simulink model "projekt"  (R2021b)
settings: Solver=FixedStepAuto  StartTime=0.0  StopTime=Inf  RelTol=1e-3  EnableMultiTasking=on
libraries: c2837xDlib x30
settings Model: ExtModeTrigDuration=8  Creator=gabrys  LastModifiedBy=gabrys
settings SolverCC: AutoInsertRateTranBlk=on
settings OptimizationCC: DefaultUnderspecifiedDataType=single  EnhancedBackFolding=on  PassReuseOutputArgsAs=Individual arguments  MaxStackSize=1024  OptimizeBlockOrder=speed  DifferentSizesBufferReuse=on  OptimizationCustomize=off  DenormalBehavior=FlushToZero  EfficientTunableParamExpr=on
settings DebuggingCC: ParameterTunabilityLossMsg=error
settings HardwareCC: ProdBitPerChar=16  ProdBitPerInt=16  ProdBitPerPointer=32  ProdBitPerSizeT=32  ProdBitPerPtrDiffT=32  ProdLargestAtomicInteger=Integer  ProdLargestAtomicFloat=None  ProdWordSize=16  ProdLongLongMode=on  ProdHWDeviceType=Texas Instruments->C2000
settings ModelReferenceCC: ModelReferenceNumInstancesAllowed=Single
settings SFSimCC: MATLABDynamicMemAlloc=off
settings RTWCC: Description=Embedded Coder  SystemTargetFile=ert.tlc  HardwareBoard=TI Delfino F28379D LaunchPad  TemplateMakefile=ert_default_tmf  Toolchain=Texas Instruments Code Composer Studio (C2000)
settings CodeAppCC: ForceParamTrailComments=on  IgnoreCustomStorageClasses=off  OperatorAnnotations=on  SimulinkDataObjDesc=on  SFDataObjDesc=on  InsertBlockDesc=on
settings ERTTargetCC: CodeReplacementLibrary=TI C28x  ExtModeTransport=4  ExtModeStaticAlloc=on  ExtModeMexFile=ext_xcp  ExtModeIntrfLevel=Level2 - Open

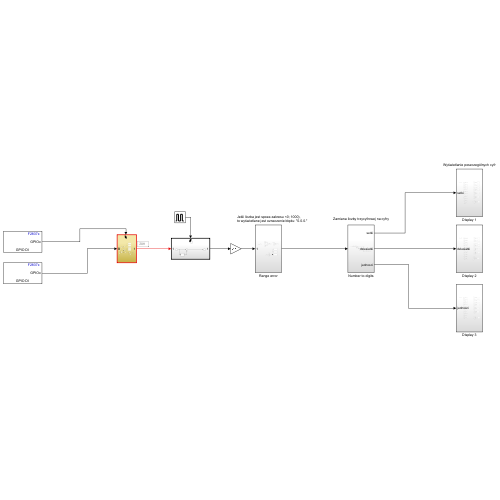
[thumbnail: Simulink's stored preview of the top-level diagram]
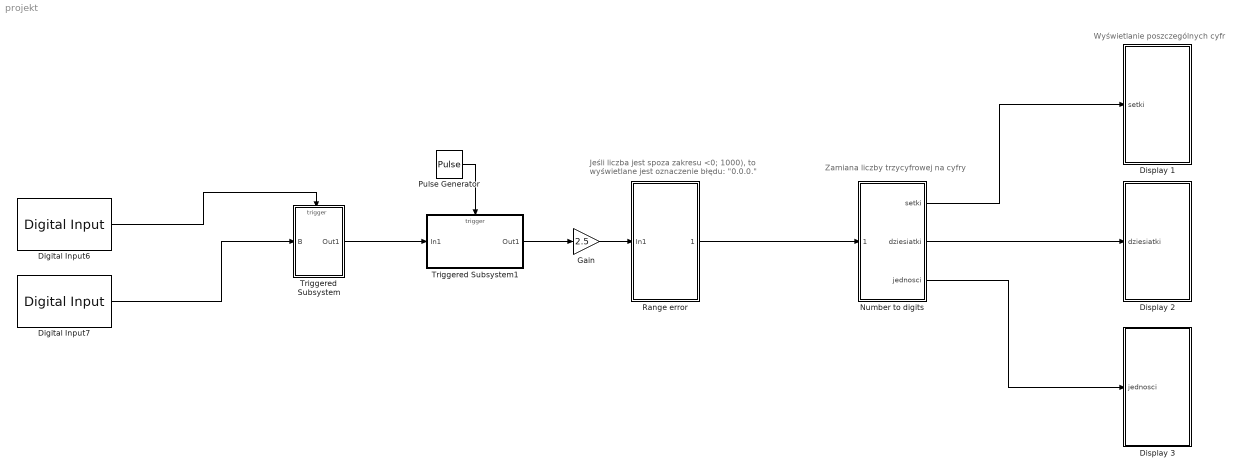
== system projekt ==
  note: Jeśli liczba jest spoza zakresu <0; 1000),
      | to wyświetlane jest oznaczenie błędu: "0.0.0."
  note: Wyświetlanie poszczególnych cyfr
  note: Zamiana liczby trzycyfrowej na cyfry
  Digital Input6 : c2837xDlib/Digital Input  GPIO_Number=GPIO128~GPIO135  GPIO_Bit0=off  GPIO_Bit1=off  GPIO_Bit2=on  GPIO_Bit3=off  GPIO_Bit4=off  GPIO_Bit5=off  GPIO_Bit6=off  GPIO_Bit7=off  sampleTime=0.01  dataType=auto  GPIO_Bit0_Qualification=Sync to SYSCLKOUT  GPIO_Bit1_Qualification=Sync to SYSCLKOUT  GPIO_Bit2_Qualification=Sync to SYSCLKOUT  GPIO_Bit3_Qualification=Sync to SYSCLKOUT  GPIO_Bit4_Qualification=Sync to SYSCLKOUT  GPIO_Bit5_Qualification=Sync to SYSCLKOUT  GPIO_Bit6_Qualification=Sync to SYSCLKOUT  GPIO_Bit7_Qualification=Sync to SYSCLKOUT  Qualification_Period=-1
      settings: SourceProductBaseCode=TIC2000
  Digital Input7 : c2837xDlib/Digital Input  GPIO_Number=GPIO128~GPIO135  GPIO_Bit0=off  GPIO_Bit1=off  GPIO_Bit2=off  GPIO_Bit3=on  GPIO_Bit4=off  GPIO_Bit5=off  GPIO_Bit6=off  GPIO_Bit7=off  sampleTime=0.01  dataType=auto  GPIO_Bit0_Qualification=Sync to SYSCLKOUT  GPIO_Bit1_Qualification=Sync to SYSCLKOUT  GPIO_Bit2_Qualification=Sync to SYSCLKOUT  GPIO_Bit3_Qualification=Sync to SYSCLKOUT  GPIO_Bit4_Qualification=Sync to SYSCLKOUT  GPIO_Bit5_Qualification=Sync to SYSCLKOUT  GPIO_Bit6_Qualification=Sync to SYSCLKOUT  GPIO_Bit7_Qualification=Sync to SYSCLKOUT  Qualification_Period=-1
      settings: SourceProductBaseCode=TIC2000
  Display 1 : Subsystem
  Display 2 : Subsystem
  Display 3 : Subsystem
  Gain : Gain  Gain=2.5
  Number to digits : Subsystem
  Pulse Generator : DiscretePulseGenerator  PulseType=Time based  Period=1  PulseWidth=50
  Range error : Subsystem
  Triggered Subsystem : Subsystem  TreatAsAtomicUnit=on
  Triggered Subsystem1 : Subsystem  TreatAsAtomicUnit=on
  wires:
  Number to digits/3(jednosci) -> Display 3/1(jednosci)
  Range error/1(" ") -> Number to digits/1(" ")
  Number to digits/2(dziesiatki) -> Display 2/1(dziesiatki)
  Number to digits/1(setki) -> Display 1/1(setki)
  Digital Input7/1 -> Triggered Subsystem/1(B)
  Digital Input6/1 -> Triggered Subsystem/Trigger
  Pulse Generator/1 -> Triggered Subsystem1/Trigger
  Triggered Subsystem1/1(Out1) -> Gain/1
  Gain/1 -> Range error/1(In1)
  Triggered Subsystem/1(Out1) -> Triggered Subsystem1/1(In1)

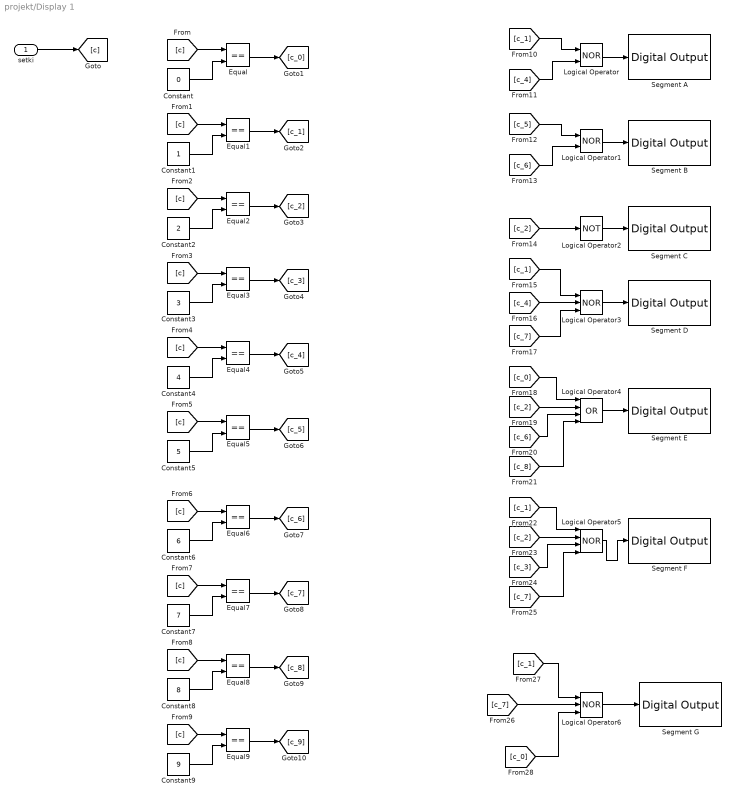
== system projekt/Display 1 ==
  setki : Inport
  Constant : Constant  Value=0
  Constant1 : Constant
  Constant2 : Constant  Value=2
  Constant3 : Constant  Value=3
  Constant4 : Constant  Value=4
  Constant5 : Constant  Value=5
  Constant6 : Constant  Value=6
  Constant7 : Constant  Value=7
  Constant8 : Constant  Value=8
  Constant9 : Constant  Value=9
  Equal{,1..9} (10 alike) : RelationalOperator  Operator===  OutDataTypeStr=boolean  RndMeth=Simplest
  Logical Operator : Logic  Operator=NOR  AllPortsSameDT=off  OutDataTypeStr=boolean
  Logical Operator1 : Logic  Operator=NOR  AllPortsSameDT=off  OutDataTypeStr=boolean
  Logical Operator2 : Logic  Operator=NOT  AllPortsSameDT=off  OutDataTypeStr=boolean
  Logical Operator3 : Logic  Operator=NOR  Inputs=3  AllPortsSameDT=off  OutDataTypeStr=boolean
  Logical Operator4 : Logic  Operator=OR  Inputs=4  AllPortsSameDT=off  OutDataTypeStr=boolean
  Logical Operator5 : Logic  Operator=NOR  Inputs=4  AllPortsSameDT=off  OutDataTypeStr=boolean
  Logical Operator6 : Logic  Operator=NOR  Inputs=3  AllPortsSameDT=off  OutDataTypeStr=boolean
  Segment A : c2837xDlib/Digital Output  GPIO_Number=GPIO0~GPIO7  GPIO_Bit0=off  GPIO_BIT0_Toggle=off  GPIO_Bit1=on  GPIO_BIT1_Toggle=off  GPIO_Bit2=off  GPIO_BIT2_Toggle=off  GPIO_Bit3=off  GPIO_BIT3_Toggle=off  GPIO_Bit4=off  GPIO_BIT4_Toggle=off  GPIO_Bit5=off  GPIO_BIT5_Toggle=off  GPIO_Bit6=off  GPIO_BIT6_Toggle=off  GPIO_Bit7=off  GPIO_BIT7_Toggle=off
      settings: SourceProductBaseCode=TIC2000
  Segment B : c2837xDlib/Digital Output  GPIO_Number=GPIO120~GPIO127  GPIO_Bit0=off  GPIO_BIT0_Toggle=off  GPIO_Bit1=off  GPIO_BIT1_Toggle=off  GPIO_Bit2=off  GPIO_BIT2_Toggle=off  GPIO_Bit3=on  GPIO_BIT3_Toggle=off  GPIO_Bit4=off  GPIO_BIT4_Toggle=off  GPIO_Bit5=off  GPIO_BIT5_Toggle=off  GPIO_Bit6=off  GPIO_BIT6_Toggle=off  GPIO_Bit7=off  GPIO_BIT7_Toggle=off
      settings: SourceProductBaseCode=TIC2000
  Segment C : c2837xDlib/Digital Output  GPIO_Number=GPIO16~GPIO23  GPIO_Bit0=off  GPIO_BIT0_Toggle=off  GPIO_Bit1=off  GPIO_BIT1_Toggle=off  GPIO_Bit2=on  GPIO_BIT2_Toggle=off  GPIO_Bit3=off  GPIO_BIT3_Toggle=off  GPIO_Bit4=off  GPIO_BIT4_Toggle=off  GPIO_Bit5=off  GPIO_BIT5_Toggle=off  GPIO_Bit6=off  GPIO_BIT6_Toggle=off  GPIO_Bit7=off  GPIO_BIT7_Toggle=off
      settings: SourceProductBaseCode=TIC2000
  Segment D : c2837xDlib/Digital Output  GPIO_Number=GPIO16~GPIO23  GPIO_Bit0=off  GPIO_BIT0_Toggle=off  GPIO_Bit1=off  GPIO_BIT1_Toggle=off  GPIO_Bit2=off  GPIO_BIT2_Toggle=off  GPIO_Bit3=on  GPIO_BIT3_Toggle=off  GPIO_Bit4=off  GPIO_BIT4_Toggle=off  GPIO_Bit5=off  GPIO_BIT5_Toggle=off  GPIO_Bit6=off  GPIO_BIT6_Toggle=off  GPIO_Bit7=off  GPIO_BIT7_Toggle=off
      settings: SourceProductBaseCode=TIC2000
  Segment E : c2837xDlib/Digital Output  GPIO_Number=GPIO32~GPIO39  GPIO_Bit0=on  GPIO_BIT0_Toggle=off  GPIO_Bit1=off  GPIO_BIT1_Toggle=off  GPIO_Bit2=off  GPIO_BIT2_Toggle=off  GPIO_Bit3=off  GPIO_BIT3_Toggle=off  GPIO_Bit4=off  GPIO_BIT4_Toggle=off  GPIO_Bit5=off  GPIO_BIT5_Toggle=off  GPIO_Bit6=off  GPIO_BIT6_Toggle=off  GPIO_Bit7=off  GPIO_BIT7_Toggle=off
      settings: SourceProductBaseCode=TIC2000
  Segment F : c2837xDlib/Digital Output  GPIO_Number=GPIO56~GPIO63  GPIO_Bit0=off  GPIO_BIT0_Toggle=off  GPIO_Bit1=off  GPIO_BIT1_Toggle=off  GPIO_Bit2=off  GPIO_BIT2_Toggle=off  GPIO_Bit3=off  GPIO_BIT3_Toggle=off  GPIO_Bit4=off  GPIO_BIT4_Toggle=off  GPIO_Bit5=on  GPIO_BIT5_Toggle=off  GPIO_Bit6=off  GPIO_BIT6_Toggle=off  GPIO_Bit7=off  GPIO_BIT7_Toggle=off
      settings: SourceProductBaseCode=TIC2000
  Segment G : c2837xDlib/Digital Output  GPIO_Number=GPIO0~GPIO7  GPIO_Bit0=on  GPIO_BIT0_Toggle=off  GPIO_Bit1=off  GPIO_BIT1_Toggle=off  GPIO_Bit2=off  GPIO_BIT2_Toggle=off  GPIO_Bit3=off  GPIO_BIT3_Toggle=off  GPIO_Bit4=off  GPIO_BIT4_Toggle=off  GPIO_Bit5=off  GPIO_BIT5_Toggle=off  GPIO_Bit6=off  GPIO_BIT6_Toggle=off  GPIO_Bit7=off  GPIO_BIT7_Toggle=off
      settings: SourceProductBaseCode=TIC2000
  wires:
  setki/1 -> [c]
  [c] -> Equal/1
  Constant/1 -> Equal/2
  Equal/1 -> [c_0]
  Constant1/1 -> Equal1/2
  [c] -> Equal1/1
  Equal1/1 -> [c_1]
  Constant2/1 -> Equal2/2
  [c] -> Equal2/1
  Equal2/1 -> [c_2]
  Equal4/1 -> [c_4]
  Constant4/1 -> Equal4/2
  [c] -> Equal4/1
  [c] -> Equal5/1
  Constant5/1 -> Equal5/2
  Constant3/1 -> Equal3/2
  [c] -> Equal3/1
  Equal3/1 -> [c_3]
  Equal5/1 -> [c_5]
  Equal6/1 -> [c_6]
  Constant6/1 -> Equal6/2
  Equal7/1 -> [c_7]
  [c] -> Equal7/1
  [c] -> Equal6/1
  Constant7/1 -> Equal7/2
  [c] -> Equal8/1
  Constant8/1 -> Equal8/2
  [c] -> Equal9/1
  Constant9/1 -> Equal9/2
  Equal8/1 -> [c_8]
  Equal9/1 -> [c_9]
  Logical Operator/1 -> Segment A/1
  [c_1] -> Logical Operator/1
  [c_4] -> Logical Operator/2
  [c_6] -> Logical Operator1/2
  Logical Operator1/1 -> Segment B/1
  [c_5] -> Logical Operator1/1
  [c_2] -> Logical Operator2/1
  Logical Operator2/1 -> Segment C/1
  [c_1] -> Logical Operator3/1
  Logical Operator3/1 -> Segment D/1
  [c_4] -> Logical Operator3/2
  [c_7] -> Logical Operator3/3
  [c_6] -> Logical Operator4/3
  [c_2] -> Logical Operator4/2
  Logical Operator4/1 -> Segment E/1
  [c_0] -> Logical Operator4/1
  [c_8] -> Logical Operator4/4
  [c_2] -> Logical Operator5/2
  [c_1] -> Logical Operator5/1
  Logical Operator5/1 -> Segment F/1
  [c_3] -> Logical Operator5/3
  [c_7] -> Logical Operator5/4
  [c_7] -> Logical Operator6/2
  Logical Operator6/1 -> Segment G/1
  [c_1] -> Logical Operator6/1
  [c_0] -> Logical Operator6/3

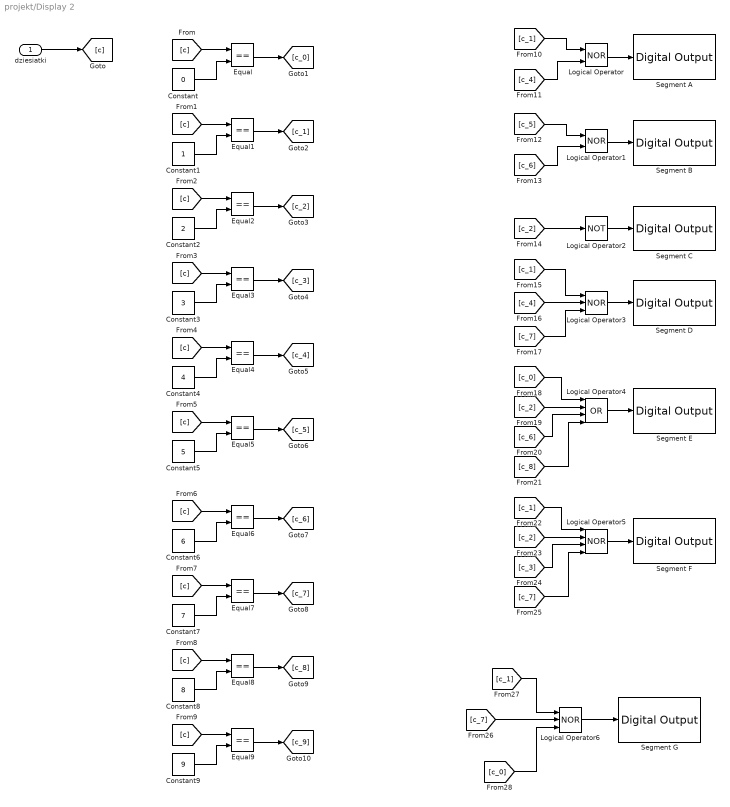
== system projekt/Display 2 ==
  dziesiatki : Inport
  Constant : Constant  Value=0
  Constant1 : Constant
  Constant2 : Constant  Value=2
  Constant3 : Constant  Value=3
  Constant4 : Constant  Value=4
  Constant5 : Constant  Value=5
  Constant6 : Constant  Value=6
  Constant7 : Constant  Value=7
  Constant8 : Constant  Value=8
  Constant9 : Constant  Value=9
  Equal{,1..9} (10 alike) : RelationalOperator  Operator===  OutDataTypeStr=boolean  RndMeth=Simplest
  Logical Operator : Logic  Operator=NOR  AllPortsSameDT=off  OutDataTypeStr=boolean
  Logical Operator1 : Logic  Operator=NOR  AllPortsSameDT=off  OutDataTypeStr=boolean
  Logical Operator2 : Logic  Operator=NOT  AllPortsSameDT=off  OutDataTypeStr=boolean
  Logical Operator3 : Logic  Operator=NOR  Inputs=3  AllPortsSameDT=off  OutDataTypeStr=boolean
  Logical Operator4 : Logic  Operator=OR  Inputs=4  AllPortsSameDT=off  OutDataTypeStr=boolean
  Logical Operator5 : Logic  Operator=NOR  Inputs=4  AllPortsSameDT=off  OutDataTypeStr=boolean
  Logical Operator6 : Logic  Operator=NOR  Inputs=3  AllPortsSameDT=off  OutDataTypeStr=boolean
  Segment A : c2837xDlib/Digital Output  GPIO_Number=GPIO120~GPIO127  GPIO_Bit0=off  GPIO_BIT0_Toggle=off  GPIO_Bit1=off  GPIO_BIT1_Toggle=off  GPIO_Bit2=on  GPIO_BIT2_Toggle=off  GPIO_Bit3=off  GPIO_BIT3_Toggle=off  GPIO_Bit4=off  GPIO_BIT4_Toggle=off  GPIO_Bit5=off  GPIO_BIT5_Toggle=off  GPIO_Bit6=off  GPIO_BIT6_Toggle=off  GPIO_Bit7=off  GPIO_BIT7_Toggle=off
      settings: SourceProductBaseCode=TIC2000
  Segment B : c2837xDlib/Digital Output  GPIO_Number=GPIO0~GPIO7  GPIO_Bit0=off  GPIO_BIT0_Toggle=off  GPIO_Bit1=off  GPIO_BIT1_Toggle=off  GPIO_Bit2=off  GPIO_BIT2_Toggle=off  GPIO_Bit3=off  GPIO_BIT3_Toggle=off  GPIO_Bit4=on  GPIO_BIT4_Toggle=off  GPIO_Bit5=off  GPIO_BIT5_Toggle=off  GPIO_Bit6=off  GPIO_BIT6_Toggle=off  GPIO_Bit7=off  GPIO_BIT7_Toggle=off
      settings: SourceProductBaseCode=TIC2000
  Segment C : c2837xDlib/Digital Output  GPIO_Number=GPIO16~GPIO23  GPIO_Bit0=off  GPIO_BIT0_Toggle=off  GPIO_Bit1=off  GPIO_BIT1_Toggle=off  GPIO_Bit2=off  GPIO_BIT2_Toggle=off  GPIO_Bit3=off  GPIO_BIT3_Toggle=off  GPIO_Bit4=off  GPIO_BIT4_Toggle=off  GPIO_Bit5=off  GPIO_BIT5_Toggle=off  GPIO_Bit6=on  GPIO_BIT6_Toggle=off  GPIO_Bit7=off  GPIO_BIT7_Toggle=off
      settings: SourceProductBaseCode=TIC2000
  Segment D : c2837xDlib/Digital Output  GPIO_Number=GPIO56~GPIO63  GPIO_Bit0=off  GPIO_BIT0_Toggle=off  GPIO_Bit1=off  GPIO_BIT1_Toggle=off  GPIO_Bit2=off  GPIO_BIT2_Toggle=off  GPIO_Bit3=off  GPIO_BIT3_Toggle=off  GPIO_Bit4=on  GPIO_BIT4_Toggle=off  GPIO_Bit5=off  GPIO_BIT5_Toggle=off  GPIO_Bit6=off  GPIO_BIT6_Toggle=off  GPIO_Bit7=off  GPIO_BIT7_Toggle=off
      settings: SourceProductBaseCode=TIC2000
  Segment E : c2837xDlib/Digital Output  GPIO_Number=GPIO104~GPIO111  GPIO_Bit0=off  GPIO_BIT0_Toggle=off  GPIO_Bit1=off  GPIO_BIT1_Toggle=off  GPIO_Bit2=off  GPIO_BIT2_Toggle=off  GPIO_Bit3=off  GPIO_BIT3_Toggle=off  GPIO_Bit4=off  GPIO_BIT4_Toggle=off  GPIO_Bit5=off  GPIO_BIT5_Toggle=off  GPIO_Bit6=off  GPIO_BIT6_Toggle=off  GPIO_Bit7=on  GPIO_BIT7_Toggle=off
      settings: SourceProductBaseCode=TIC2000
  Segment F : c2837xDlib/Digital Output  GPIO_Number=GPIO0~GPIO7  GPIO_Bit0=off  GPIO_BIT0_Toggle=off  GPIO_Bit1=off  GPIO_BIT1_Toggle=off  GPIO_Bit2=off  GPIO_BIT2_Toggle=off  GPIO_Bit3=on  GPIO_BIT3_Toggle=off  GPIO_Bit4=off  GPIO_BIT4_Toggle=off  GPIO_Bit5=off  GPIO_BIT5_Toggle=off  GPIO_Bit6=off  GPIO_BIT6_Toggle=off  GPIO_Bit7=off  GPIO_BIT7_Toggle=off
      settings: SourceProductBaseCode=TIC2000
  Segment G : c2837xDlib/Digital Output  GPIO_Number=GPIO0~GPIO7  GPIO_Bit0=off  GPIO_BIT0_Toggle=off  GPIO_Bit1=off  GPIO_BIT1_Toggle=off  GPIO_Bit2=on  GPIO_BIT2_Toggle=off  GPIO_Bit3=off  GPIO_BIT3_Toggle=off  GPIO_Bit4=off  GPIO_BIT4_Toggle=off  GPIO_Bit5=off  GPIO_BIT5_Toggle=off  GPIO_Bit6=off  GPIO_BIT6_Toggle=off  GPIO_Bit7=off  GPIO_BIT7_Toggle=off
      settings: SourceProductBaseCode=TIC2000
  wires:
  dziesiatki/1 -> [c]
  [c] -> Equal/1
  Constant/1 -> Equal/2
  Equal/1 -> [c_0]
  Constant1/1 -> Equal1/2
  [c] -> Equal1/1
  Equal1/1 -> [c_1]
  Constant2/1 -> Equal2/2
  [c] -> Equal2/1
  Equal2/1 -> [c_2]
  Equal4/1 -> [c_4]
  Constant4/1 -> Equal4/2
  [c] -> Equal4/1
  [c] -> Equal5/1
  Constant5/1 -> Equal5/2
  Constant3/1 -> Equal3/2
  [c] -> Equal3/1
  Equal3/1 -> [c_3]
  Equal5/1 -> [c_5]
  Equal6/1 -> [c_6]
  Constant6/1 -> Equal6/2
  Equal7/1 -> [c_7]
  [c] -> Equal7/1
  [c] -> Equal6/1
  Constant7/1 -> Equal7/2
  [c] -> Equal8/1
  Constant8/1 -> Equal8/2
  [c] -> Equal9/1
  Constant9/1 -> Equal9/2
  Equal8/1 -> [c_8]
  Equal9/1 -> [c_9]
  Logical Operator/1 -> Segment A/1
  [c_1] -> Logical Operator/1
  [c_4] -> Logical Operator/2
  [c_6] -> Logical Operator1/2
  Logical Operator1/1 -> Segment B/1
  [c_5] -> Logical Operator1/1
  [c_2] -> Logical Operator2/1
  Logical Operator2/1 -> Segment C/1
  [c_1] -> Logical Operator3/1
  Logical Operator3/1 -> Segment D/1
  [c_4] -> Logical Operator3/2
  [c_7] -> Logical Operator3/3
  [c_6] -> Logical Operator4/3
  [c_2] -> Logical Operator4/2
  Logical Operator4/1 -> Segment E/1
  [c_0] -> Logical Operator4/1
  [c_8] -> Logical Operator4/4
  [c_2] -> Logical Operator5/2
  [c_1] -> Logical Operator5/1
  Logical Operator5/1 -> Segment F/1
  [c_3] -> Logical Operator5/3
  [c_7] -> Logical Operator5/4
  [c_7] -> Logical Operator6/2
  Logical Operator6/1 -> Segment G/1
  [c_1] -> Logical Operator6/1
  [c_0] -> Logical Operator6/3

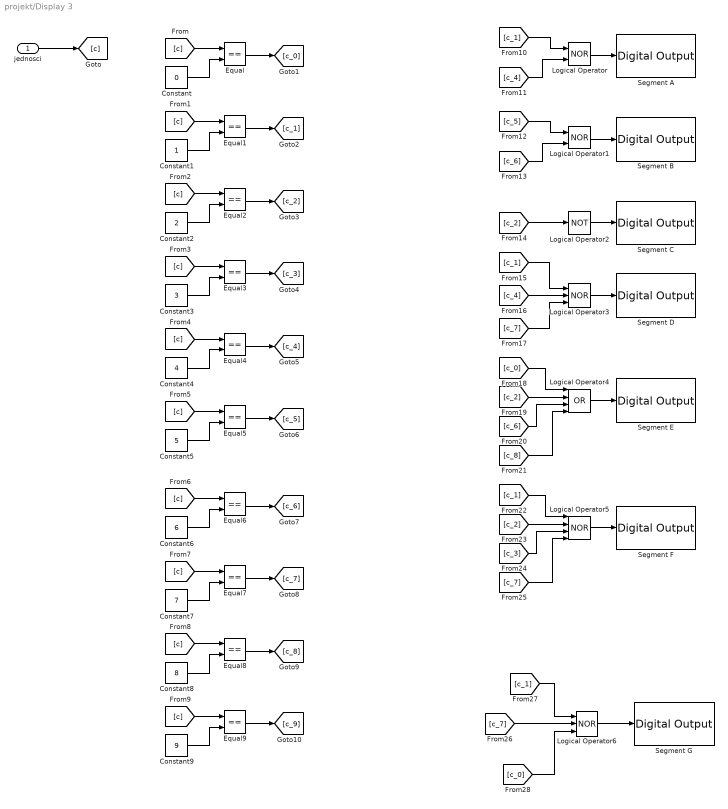
== system projekt/Display 3 ==
  jednosci : Inport
  Constant : Constant  Value=0
  Constant1 : Constant
  Constant2 : Constant  Value=2
  Constant3 : Constant  Value=3
  Constant4 : Constant  Value=4
  Constant5 : Constant  Value=5
  Constant6 : Constant  Value=6
  Constant7 : Constant  Value=7
  Constant8 : Constant  Value=8
  Constant9 : Constant  Value=9
  Equal{,1..9} (10 alike) : RelationalOperator  Operator===  OutDataTypeStr=boolean  RndMeth=Simplest
  Logical Operator : Logic  Operator=NOR  AllPortsSameDT=off  OutDataTypeStr=boolean
  Logical Operator1 : Logic  Operator=NOR  AllPortsSameDT=off  OutDataTypeStr=boolean
  Logical Operator2 : Logic  Operator=NOT  AllPortsSameDT=off  OutDataTypeStr=boolean
  Logical Operator3 : Logic  Operator=NOR  Inputs=3  AllPortsSameDT=off  OutDataTypeStr=boolean
  Logical Operator4 : Logic  Operator=OR  Inputs=4  AllPortsSameDT=off  OutDataTypeStr=boolean
  Logical Operator5 : Logic  Operator=NOR  Inputs=4  AllPortsSameDT=off  OutDataTypeStr=boolean
  Logical Operator6 : Logic  Operator=NOR  Inputs=3  AllPortsSameDT=off  OutDataTypeStr=boolean
  Segment A : c2837xDlib/Digital Output  GPIO_Number=GPIO24~GPIO31  GPIO_Bit0=on  GPIO_BIT0_Toggle=off  GPIO_Bit1=off  GPIO_BIT1_Toggle=off  GPIO_Bit2=off  GPIO_BIT2_Toggle=off  GPIO_Bit3=off  GPIO_BIT3_Toggle=off  GPIO_Bit4=off  GPIO_BIT4_Toggle=off  GPIO_Bit5=off  GPIO_BIT5_Toggle=off  GPIO_Bit6=off  GPIO_BIT6_Toggle=off  GPIO_Bit7=off  GPIO_BIT7_Toggle=off
      settings: SourceProductBaseCode=TIC2000
  Segment B : c2837xDlib/Digital Output  GPIO_Number=GPIO16~GPIO23  GPIO_Bit0=on  GPIO_BIT0_Toggle=off  GPIO_Bit1=off  GPIO_BIT1_Toggle=off  GPIO_Bit2=off  GPIO_BIT2_Toggle=off  GPIO_Bit3=off  GPIO_BIT3_Toggle=off  GPIO_Bit4=off  GPIO_BIT4_Toggle=off  GPIO_Bit5=off  GPIO_BIT5_Toggle=off  GPIO_Bit6=off  GPIO_BIT6_Toggle=off  GPIO_Bit7=off  GPIO_BIT7_Toggle=off
      settings: SourceProductBaseCode=TIC2000
  Segment C : c2837xDlib/Digital Output  GPIO_Number=GPIO136~GPIO143  GPIO_Bit0=off  GPIO_BIT0_Toggle=off  GPIO_Bit1=off  GPIO_BIT1_Toggle=off  GPIO_Bit2=off  GPIO_BIT2_Toggle=off  GPIO_Bit3=on  GPIO_BIT3_Toggle=off  GPIO_Bit4=off  GPIO_BIT4_Toggle=off  GPIO_Bit5=off  GPIO_BIT5_Toggle=off  GPIO_Bit6=off  GPIO_BIT6_Toggle=off  GPIO_Bit7=off  GPIO_BIT7_Toggle=off
      settings: SourceProductBaseCode=TIC2000
  Segment D : c2837xDlib/Digital Output  GPIO_Number=GPIO56~GPIO63  GPIO_Bit0=on  GPIO_BIT0_Toggle=off  GPIO_Bit1=off  GPIO_BIT1_Toggle=off  GPIO_Bit2=off  GPIO_BIT2_Toggle=off  GPIO_Bit3=off  GPIO_BIT3_Toggle=off  GPIO_Bit4=off  GPIO_BIT4_Toggle=off  GPIO_Bit5=off  GPIO_BIT5_Toggle=off  GPIO_Bit6=off  GPIO_BIT6_Toggle=off  GPIO_Bit7=off  GPIO_BIT7_Toggle=off
      settings: SourceProductBaseCode=TIC2000
  Segment E : c2837xDlib/Digital Output  GPIO_Number=GPIO104~GPIO111  GPIO_Bit0=on  GPIO_BIT0_Toggle=off  GPIO_Bit1=off  GPIO_BIT1_Toggle=off  GPIO_Bit2=off  GPIO_BIT2_Toggle=off  GPIO_Bit3=off  GPIO_BIT3_Toggle=off  GPIO_Bit4=off  GPIO_BIT4_Toggle=off  GPIO_Bit5=off  GPIO_BIT5_Toggle=off  GPIO_Bit6=off  GPIO_BIT6_Toggle=off  GPIO_Bit7=off  GPIO_BIT7_Toggle=off
      settings: SourceProductBaseCode=TIC2000
  Segment F : c2837xDlib/Digital Output  GPIO_Number=GPIO56~GPIO63  GPIO_Bit0=off  GPIO_BIT0_Toggle=off  GPIO_Bit1=off  GPIO_BIT1_Toggle=off  GPIO_Bit2=on  GPIO_BIT2_Toggle=off  GPIO_Bit3=off  GPIO_BIT3_Toggle=off  GPIO_Bit4=off  GPIO_BIT4_Toggle=off  GPIO_Bit5=off  GPIO_BIT5_Toggle=off  GPIO_Bit6=off  GPIO_BIT6_Toggle=off  GPIO_Bit7=off  GPIO_BIT7_Toggle=off
      settings: SourceProductBaseCode=TIC2000
  Segment G : c2837xDlib/Digital Output  GPIO_Number=GPIO0~GPIO7  GPIO_Bit0=off  GPIO_BIT0_Toggle=off  GPIO_Bit1=off  GPIO_BIT1_Toggle=off  GPIO_Bit2=off  GPIO_BIT2_Toggle=off  GPIO_Bit3=off  GPIO_BIT3_Toggle=off  GPIO_Bit4=off  GPIO_BIT4_Toggle=off  GPIO_Bit5=on  GPIO_BIT5_Toggle=off  GPIO_Bit6=off  GPIO_BIT6_Toggle=off  GPIO_Bit7=off  GPIO_BIT7_Toggle=off
      settings: SourceProductBaseCode=TIC2000
  wires:
  jednosci/1 -> [c]
  [c] -> Equal/1
  Constant/1 -> Equal/2
  Equal/1 -> [c_0]
  Constant1/1 -> Equal1/2
  [c] -> Equal1/1
  Equal1/1 -> [c_1]
  Constant2/1 -> Equal2/2
  [c] -> Equal2/1
  Equal2/1 -> [c_2]
  Equal4/1 -> [c_4]
  Constant4/1 -> Equal4/2
  [c] -> Equal4/1
  [c] -> Equal5/1
  Constant5/1 -> Equal5/2
  Constant3/1 -> Equal3/2
  [c] -> Equal3/1
  Equal3/1 -> [c_3]
  Equal5/1 -> [c_5]
  Equal6/1 -> [c_6]
  Constant6/1 -> Equal6/2
  Equal7/1 -> [c_7]
  [c] -> Equal7/1
  [c] -> Equal6/1
  Constant7/1 -> Equal7/2
  [c] -> Equal8/1
  Constant8/1 -> Equal8/2
  [c] -> Equal9/1
  Constant9/1 -> Equal9/2
  Equal8/1 -> [c_8]
  Equal9/1 -> [c_9]
  Logical Operator/1 -> Segment A/1
  [c_1] -> Logical Operator/1
  [c_4] -> Logical Operator/2
  [c_6] -> Logical Operator1/2
  Logical Operator1/1 -> Segment B/1
  [c_5] -> Logical Operator1/1
  [c_2] -> Logical Operator2/1
  Logical Operator2/1 -> Segment C/1
  [c_1] -> Logical Operator3/1
  Logical Operator3/1 -> Segment D/1
  [c_4] -> Logical Operator3/2
  [c_7] -> Logical Operator3/3
  [c_6] -> Logical Operator4/3
  [c_2] -> Logical Operator4/2
  Logical Operator4/1 -> Segment E/1
  [c_0] -> Logical Operator4/1
  [c_8] -> Logical Operator4/4
  [c_2] -> Logical Operator5/2
  [c_1] -> Logical Operator5/1
  Logical Operator5/1 -> Segment F/1
  [c_3] -> Logical Operator5/3
  [c_7] -> Logical Operator5/4
  Logical Operator6/1 -> Segment G/1
  [c_1] -> Logical Operator6/1
  [c_7] -> Logical Operator6/2
  [c_0] -> Logical Operator6/3

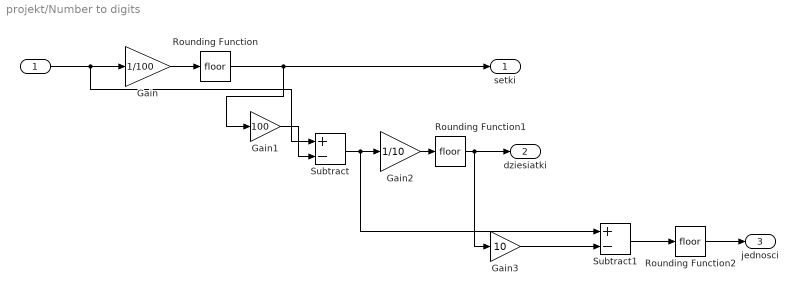
== system projekt/Number to digits ==
  " " : Inport
  Gain : Gain  Gain=1/100
  Gain1 : Gain  Gain=100
  Gain2 : Gain  Gain=1/10
  Gain3 : Gain  Gain=10
  Rounding Function : Rounding
  Rounding Function1 : Rounding
  Rounding Function2 : Rounding
  Subtract : Sum  Inputs=+-
  Subtract1 : Sum  Inputs=+-
  setki : Outport
  dziesiatki : Outport  Port=2
  jednosci : Outport  Port=3
  wires:
  " "/1 -> Subtract/1, Gain/1
  Gain/1 -> Rounding Function/1
  Rounding Function/1 -> Gain1/1, setki/1
  Gain1/1 -> Subtract/2
  Gain2/1 -> Rounding Function1/1
  Rounding Function1/1 -> Gain3/1, dziesiatki/1
  Subtract/1 -> Subtract1/1, Gain2/1
  Gain3/1 -> Subtract1/2
  Subtract1/1 -> Rounding Function2/1
  Rounding Function2/1 -> jednosci/1

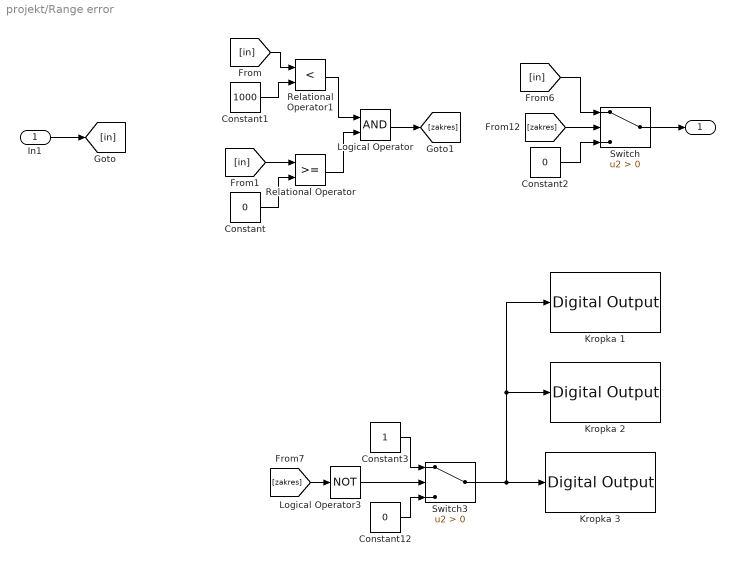
== system projekt/Range error ==
  In1 : Inport
  Constant : Constant  Value=0
  Constant1 : Constant  Value=1000
  Constant12 : Constant  Value=0
  Constant2 : Constant  Value=0
  Constant3 : Constant
  Kropka 1 : c2837xDlib/Digital Output  GPIO_Number=GPIO104~GPIO111  GPIO_Bit0=off  GPIO_BIT0_Toggle=off  GPIO_Bit1=on  GPIO_BIT1_Toggle=off  GPIO_Bit2=off  GPIO_BIT2_Toggle=off  GPIO_Bit3=off  GPIO_BIT3_Toggle=off  GPIO_Bit4=off  GPIO_BIT4_Toggle=off  GPIO_Bit5=off  GPIO_BIT5_Toggle=off  GPIO_Bit6=off  GPIO_BIT6_Toggle=off  GPIO_Bit7=off  GPIO_BIT7_Toggle=off
      settings: SourceProductBaseCode=TIC2000
  Kropka 2 : c2837xDlib/Digital Output  GPIO_Number=GPIO64~GPIO71  GPIO_Bit0=off  GPIO_BIT0_Toggle=off  GPIO_Bit1=off  GPIO_BIT1_Toggle=off  GPIO_Bit2=off  GPIO_BIT2_Toggle=off  GPIO_Bit3=on  GPIO_BIT3_Toggle=off  GPIO_Bit4=off  GPIO_BIT4_Toggle=off  GPIO_Bit5=off  GPIO_BIT5_Toggle=off  GPIO_Bit6=off  GPIO_BIT6_Toggle=off  GPIO_Bit7=off  GPIO_BIT7_Toggle=off
      settings: SourceProductBaseCode=TIC2000
  Kropka 3 : c2837xDlib/Digital Output  GPIO_Number=GPIO88~GPIO95  GPIO_Bit0=off  GPIO_BIT0_Toggle=off  GPIO_Bit1=off  GPIO_BIT1_Toggle=off  GPIO_Bit2=off  GPIO_BIT2_Toggle=off  GPIO_Bit3=off  GPIO_BIT3_Toggle=off  GPIO_Bit4=off  GPIO_BIT4_Toggle=off  GPIO_Bit5=off  GPIO_BIT5_Toggle=off  GPIO_Bit6=off  GPIO_BIT6_Toggle=off  GPIO_Bit7=on  GPIO_BIT7_Toggle=off
      settings: SourceProductBaseCode=TIC2000
  Logical Operator : Logic  AllPortsSameDT=off  OutDataTypeStr=boolean
  Logical Operator3 : Logic  Operator=NOT  AllPortsSameDT=off  OutDataTypeStr=boolean
  Relational Operator : RelationalOperator  OutDataTypeStr=boolean  RndMeth=Simplest
  Relational Operator1 : RelationalOperator  Operator=<  OutDataTypeStr=boolean  RndMeth=Simplest
  Switch : Switch  Criteria=u2 > Threshold
  Switch3 : Switch  Criteria=u2 > Threshold
  " " : Outport
  wires:
  Constant/1 -> Relational Operator/2
  Constant1/1 -> Relational Operator1/2
  In1/1 -> [in]
  [in] -> Relational Operator1/1
  [in] -> Relational Operator/1
  Relational Operator1/1 -> Logical Operator/1
  Relational Operator/1 -> Logical Operator/2
  [in] -> Switch/1
  Constant2/1 -> Switch/3
  Constant3/1 -> Switch3/1
  Constant12/1 -> Switch3/3
  Logical Operator/1 -> [zakres]
  Switch3/1 -> Kropka 2/1, Kropka 1/1, Kropka 3/1
  [zakres] -> Logical Operator3/1
  Logical Operator3/1 -> Switch3/2
  [zakres] -> Switch/2
  Switch/1 -> " "/1

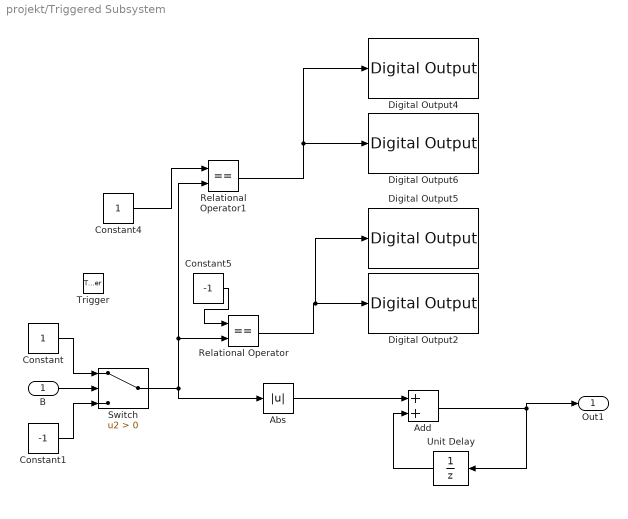
== system projekt/Triggered Subsystem ==
  B : Inport
  Trigger : TriggerPort  TriggerType=falling  VariantControl=(inherit)
  Abs : Abs
  Add : Sum
  Constant : Constant
  Constant1 : Constant  Value=-1
  Constant4 : Constant
  Constant5 : Constant  Value=-1
  Digital Output2 : c2837xDlib/Digital Output  GPIO_Number=GPIO8~GPIO15  GPIO_Bit0=off  GPIO_BIT0_Toggle=off  GPIO_Bit1=off  GPIO_BIT1_Toggle=off  GPIO_Bit2=on  GPIO_BIT2_Toggle=off  GPIO_Bit3=off  GPIO_BIT3_Toggle=off  GPIO_Bit4=off  GPIO_BIT4_Toggle=off  GPIO_Bit5=off  GPIO_BIT5_Toggle=off  GPIO_Bit6=off  GPIO_BIT6_Toggle=off  GPIO_Bit7=off  GPIO_BIT7_Toggle=off
      settings: SourceProductBaseCode=TIC2000
  Digital Output4 : c2837xDlib/Digital Output  GPIO_Number=GPIO8~GPIO15  GPIO_Bit0=off  GPIO_BIT0_Toggle=off  GPIO_Bit1=off  GPIO_BIT1_Toggle=off  GPIO_Bit2=off  GPIO_BIT2_Toggle=off  GPIO_Bit3=off  GPIO_BIT3_Toggle=off  GPIO_Bit4=off  GPIO_BIT4_Toggle=off  GPIO_Bit5=off  GPIO_BIT5_Toggle=off  GPIO_Bit6=on  GPIO_BIT6_Toggle=off  GPIO_Bit7=off  GPIO_BIT7_Toggle=off
      settings: SourceProductBaseCode=TIC2000
  Digital Output5 : c2837xDlib/Digital Output  GPIO_Number=GPIO8~GPIO15  GPIO_Bit0=off  GPIO_BIT0_Toggle=off  GPIO_Bit1=off  GPIO_BIT1_Toggle=off  GPIO_Bit2=off  GPIO_BIT2_Toggle=off  GPIO_Bit3=on  GPIO_BIT3_Toggle=off  GPIO_Bit4=off  GPIO_BIT4_Toggle=off  GPIO_Bit5=off  GPIO_BIT5_Toggle=off  GPIO_Bit6=off  GPIO_BIT6_Toggle=off  GPIO_Bit7=off  GPIO_BIT7_Toggle=off
      settings: SourceProductBaseCode=TIC2000
  Digital Output6 : c2837xDlib/Digital Output  GPIO_Number=GPIO8~GPIO15  GPIO_Bit0=off  GPIO_BIT0_Toggle=off  GPIO_Bit1=off  GPIO_BIT1_Toggle=off  GPIO_Bit2=off  GPIO_BIT2_Toggle=off  GPIO_Bit3=off  GPIO_BIT3_Toggle=off  GPIO_Bit4=off  GPIO_BIT4_Toggle=off  GPIO_Bit5=off  GPIO_BIT5_Toggle=off  GPIO_Bit6=off  GPIO_BIT6_Toggle=off  GPIO_Bit7=on  GPIO_BIT7_Toggle=off
      settings: SourceProductBaseCode=TIC2000
  Relational Operator : RelationalOperator  Operator===  OutDataTypeStr=boolean  RndMeth=Simplest
  Relational Operator1 : RelationalOperator  Operator===  OutDataTypeStr=boolean  RndMeth=Simplest
  Switch : Switch  Criteria=u2 > Threshold
  Unit Delay : UnitDelay  SampleTime=-1  HasFrameUpgradeWarning=on
  Out1 : Outport
  wires:
  Constant1/1 -> Switch/3
  B/1 -> Switch/2
  Constant/1 -> Switch/1
  Switch/1 -> Abs/1, Relational Operator1/2, Relational Operator/2
  Unit Delay/1 -> Add/2
  Add/1 -> Unit Delay/1, Out1/1
  Constant4/1 -> Relational Operator1/1
  Relational Operator/1 -> Digital Output5/1, Digital Output2/1
  Constant5/1 -> Relational Operator/1
  Relational Operator1/1 -> Digital Output4/1, Digital Output6/1
  Abs/1 -> Add/1

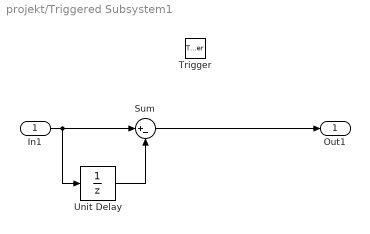
== system projekt/Triggered Subsystem1 ==
  In1 : Inport
  Trigger : TriggerPort  VariantControl=(inherit)
  Sum : Sum  Inputs=|+-
  Unit Delay : UnitDelay  SampleTime=-1  HasFrameUpgradeWarning=on
  Out1 : Outport
  wires:
  Unit Delay/1 -> Sum/2
  In1/1 -> Unit Delay/1, Sum/1
  Sum/1 -> Out1/1
